simulink model "Air_Conditioner"  (R2016b)
settings: Solver=ode23t  StartTime=0.0  StopTime=24  RelTol=1e-3  EnableMultiTasking=on
model workspace: external: MAT-File (data not in the file)
libraries: simulink x3
settings Model: Creator=jm3gonza  LastModifiedBy=Lenio
settings DataIOCC: SaveFormat=Array  SignalLoggingSaveFormat=ModelDataLogs  SaveState=on
settings OptimizationCC: ExpressionDepthLimit=2147483647  LifeSpan=inf
settings DebuggingCC: AlgebraicLoopMsg=none  UnderspecifiedInitializationDetection=Classic  MergeDetectMultiDrivingBlocksExec=none  FcnCallInpInsideContextMsg=warning  UnconnectedInputMsg=none  UnconnectedOutputMsg=none  UnconnectedLineMsg=none  StateNameClashWarn=warning  SFUnexpectedBacktrackingDiag=warning  SFNoUnconditionalDefaultTransitionDiag=warning  SFExecutionAtInitializationDiag=none
settings HardwareCC: ProdBitPerPointer=32  ProdBitPerSizeT=32  ProdBitPerPtrDiffT=32  ProdLargestAtomicFloat=None  ProdIntDivRoundTo=Undefined  ProdEndianess=Unspecified  ProdWordSize=32  ProdHWDeviceType=32-bit Generic
settings ModelReferenceCC: PropagateSignalLabelsOutOfModel=off
settings GRTTargetCC: TargetLangStandard=C89/C90 (ANSI)  GeneratePreprocessorConditionals=Disable all  CombineOutputUpdateFcns=off  GRTInterface=on
settings ConfigComp: CovMetricSettings=dw  CovHtmlReporting=on  CovSaveCumulativeToWorkspaceVar=on  CovSaveSingleToWorkspaceVar=on  CovExternalEMLEnable=off

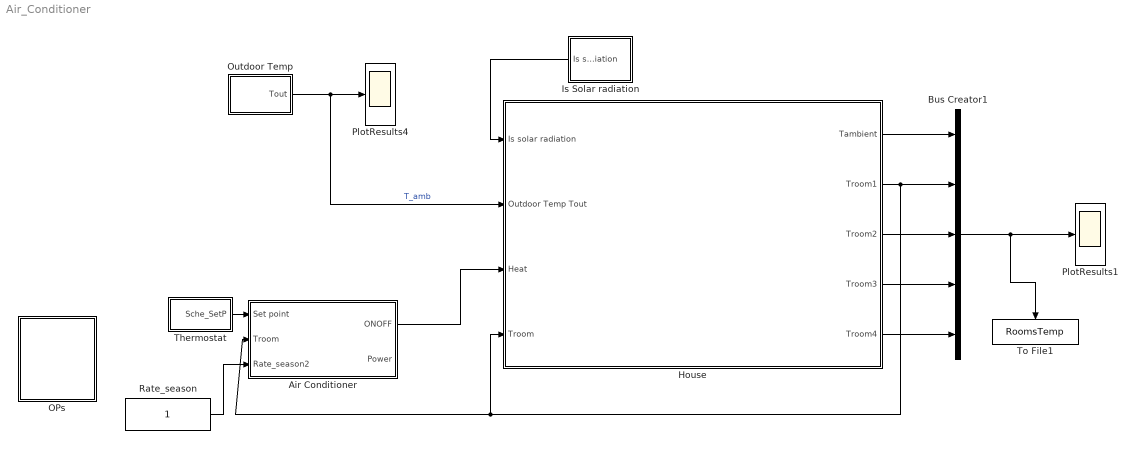
== system Air_Conditioner ==
  Air Conditioner : Subsystem
  Bus Creator1 : BusCreator  Inputs=5
  House : Subsystem
  Is Solar radiation : Subsystem
  OPs : Subsystem
  Outdoor Temp : Subsystem
  PlotResults1 : Scope
  PlotResults4 : Scope
  Rate_season : Constant
  Thermostat : Subsystem
  To File1 : ToFile  Filename=RoomsTemp  MatrixName=RoomsTemp
  wires:
  Outdoor Temp/1(Tout) -> PlotResults4/1, House/2(Outdoor Temp Tout)  "T_amb"
  House/5(Troom4) -> Bus Creator1/5
  House/1(Tambient) -> Bus Creator1/1
  House/2(Troom1) -> Bus Creator1/2, House/4(Troom), Air Conditioner/2(Troom)
  House/3(Troom2) -> Bus Creator1/3
  House/4(Troom3) -> Bus Creator1/4
  Bus Creator1/1 -> To File1/1, PlotResults1/1
  Air Conditioner/1(ONOFF) -> House/3(Heat)
  Is Solar radiation/1(Is solar radiation) -> House/1(Is solar radiation)
  Thermostat/1(Sche_SetP) -> Air Conditioner/1(Set point)
  Rate_season/1 -> Air Conditioner/3(Rate_season2)

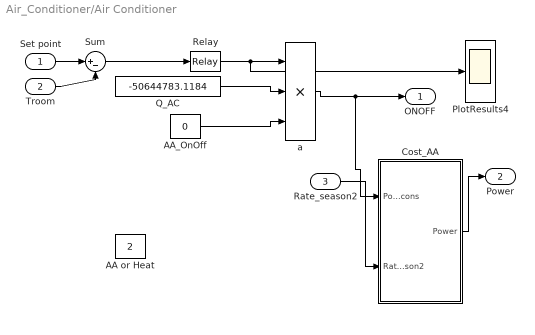
== system Air_Conditioner/Air Conditioner ==
  Set point : Inport
  Troom : Inport  Port=2
  Rate_season2 : Inport  Port=3
  AA or Heat : Constant  Value=2
  AA_OnOff : Constant  Value=0
  Cost_AA : Subsystem
  PlotResults4 : Scope
  Q_AC : Constant  Value=-50644783.1184
  Relay : Relay  OnSwitchValue=0.5  OffSwitchValue=-0.5  OnOutputValue=0  OffOutputValue=1
  Sum : Sum  Inputs=|+-  SampleTime=0  SaturateOnIntegerOverflow=on  InputSameDT=on  OutDataTypeStr=Inherit: Same as first input
  a : Product  Inputs=3  RndMeth=Zero
  ONOFF : Outport  InitialOutput=0
  Power : Outport  Port=2  InitialOutput=0
  wires:
  Set point/1 -> Sum/1
  Troom/1 -> Sum/2
  Sum/1 -> Relay/1
  Relay/1 -> a/1, PlotResults4/1
  a/1 -> ONOFF/1, Cost_AA/1(Powe_cons)
  Q_AC/1 -> a/2
  AA_OnOff/1 -> a/3
  Rate_season2/1 -> Cost_AA/2(Rate_season2)
  Cost_AA/1(Power) -> Power/1

== system Air_Conditioner/House ==
  Is solar radiation : Inport
  Outdoor Temp Tout : Inport  Port=2
  Heat : Inport  Port=3
  Troom : Inport  Port=4
  Room_1 : Subsystem
  Room_2 : Subsystem
  Room_3 : Subsystem
  Room_4 : Subsystem
  Tambient : Outport  InitialOutput=0
  Troom1 : Outport  Port=2  InitialOutput=0
  Troom2 : Outport  Port=3  InitialOutput=0
  Troom3 : Outport  Port=4  InitialOutput=0
  Troom4 : Outport  Port=5  InitialOutput=0
  wires:
  Is solar radiation/1 -> Room_1/1(Is solar radiation), Room_2/1(Is solar radiation), Room_3/1(Is solar radiation), Room_4/1(Is solar radiation)
  Outdoor Temp Tout/1 -> Room_1/2(Outdoor Temp Tout), Room_2/2(Outdoor Temp Tout), Room_3/2(Outdoor Temp Tout), Room_4/2(Outdoor Temp Tout), Tambient/1
  Heat/1 -> Room_1/3(Q_Heat), Room_2/3(Q_Heat), Room_3/3(Q_Heat), Room_4/3(Q_Heat)  "Q_Heat"
  Troom/1 -> Room_1/4(Troom), Room_2/4(Troom), Room_3/4(Troom), Room_4/4(Troom)
  Room_1/1(Room Temp Troom) -> Troom1/1
  Room_2/1(Room Temp Troom) -> Troom2/1
  Room_3/1(Room Temp Troom) -> Troom3/1
  Room_4/1(Room Temp Troom) -> Troom4/1

== system Air_Conditioner/Is Solar radiation ==
  Avg Outdoor Temp : Constant
  Outdoor Temp : simulink/Sources/Repeating Sequence Interpolated  OutValues=|  TimeValues=|  LookUpMeth=Interpolation-Use End Values  tsamp=-1  OutMin=[]  OutMax=[]  OutDataTypeStr=double  OutputDataTypeScalingMode=double  OutDataType=fixdt(0,8)  OutScaling=2^-10
      OutValues=|
      | [0
      | 0
      | 0
      | 0
      | 0
      | 0
      | 0
      | 0
      | 0
      | 0
      | 0
      | 0
      | 0
      | 0
      | 0
      | 0
      | 0
      | 0
      | 0
      | 0
      | 0
      | 12.85
      | 12.85
      | 12.85
      | 25.699
      | 38.55
      | 51.399
      | 38.55
      | 70.673
      | 70.674
      | 122.073
      | 147.772
      | 102.797
      | 237.697
      | 160.597
      | 186.273
      | 186.268
      | 173.422
      | 404.649
      | 571.658
      | 327.556
      | 411.017
      | 468.811
      | 391.717
      | 314.634
      | 237.577
      | 301.802
      | 417.367
      | 584.316
      | 449.469
      | 719.125
      | 532.917
      | 340.26
      | 199.027
      | 340.266
      | 404.503
      | 288.922
      | 314.601
      | 340.296
      | 301.769
      | 288.938
      | 263.253
      | 288.942
      | 321.049
      | 417.349
      | 327.463
      | 365.947
      | 365.936
      | 269.636
      | 224.709
      | 231.145
      | 173.362
      | 154.103
      | 147.682
      | 128.422
      | 102.737
      | 83.473
      | 70.634
      | 25.685
      | 25.686
      | 0
      | 0
      | 0
      | 0
      | 0
      | 0
      | 0
      | 0
      | 0
      | 0
      | 0
      | 0
      | 0
      | 0
      | 0
      | 0
      | ].'
      TimeValues=|
      | [         0
      |     0.1500
      |     0.3000
      |     0.4500
      |     1.0000
      |     1.1500
      |     1.3000
      |     1.4500
      |     2.0000
      |     2.1500
      |     2.3000
      |     2.4500
      |     3.0000
      |     3.1500
      |     3.3000
      |     3.4500
      |     4.0000
      |     4.1500
      |     4.3000
      |     4.4500
      |     5.0000
      |     5.1500
      |     5.3000
      |     5.4500
      |     6.0000
      |     6.1500
      |     6.3000
      |     6.4500
      |     7.0000
      |     7.1500
      |     7.3000
      |     7.4500
      |     8.0000
      |     8.1500
      |     8.3000
      |     8.4500
      |     9.0000
      |     9.1500
      |     9.3000
      |     9.4500
      |    10.0000
      |    10.1500
      |    10.3000
      |    10.4500
      |    11.0000
      |    11.1500
      |    11.3000
      |    11.4500
      |    12.0000
      |    12.1500
      |    12.3000
      |    12.4500
      |    13.0000
      |    13.1500
      |    13.3000
      |    13.4500
      |    14.0000
      |    14.1500
      |    14.3000
      |    14.4500
      |    15.0000
      |    15.1500
      |    15.3000
      |    15.4500
      |    16.0000
      |    16.1500
      |    16.3000
      |    16.4500
      |    17.0000
      |    17.1500
      |    17.3000
      |    17.4500
      |    18.0000
      |    18.1500
      |    18.3000
      |    18.4500
      |    19.0000
      |    19.1500
      |    19.3000
      |    19.4500
      |    20.0000
      |    20.1500
      |    20.3000
      |    20.4500
      |    21.0000
      |    21.1500
      |    21.3000
      |    21.4500
      |    22.0000
      |    22.1500
      |    22.3000
      |    22.4500
      |    23.0000
      |    23.1500
      |    23.3000
      |    23.4500].'
  Sum1 : Sum  Inputs=|++  SaturateOnIntegerOverflow=on  InputSameDT=on  OutDataTypeStr=Inherit: Same as first input
  Is solar radiation : Outport  InitialOutput=0
  wires:
  Avg Outdoor Temp/1 -> Sum1/1
  Outdoor Temp/1 -> Sum1/2
  Sum1/1 -> Is solar radiation/1

== system Air_Conditioner/OPs ==
  Bus Creator : BusCreator  Inputs=6
  Dishwasher_OP : Constant  Value=0
  Dryer_OP : Constant  Value=0
  EveryOP : Constant
  Lighting_OP : Constant  Value=0
  Stove_OP : Constant  Value=0
  Terminator : Terminator
  Washer_OP : Constant  Value=0
  wires:
  Lighting_OP/1 -> Bus Creator/2
  Dryer_OP/1 -> Bus Creator/3
  Dishwasher_OP/1 -> Bus Creator/4
  Washer_OP/1 -> Bus Creator/5
  EveryOP/1 -> Bus Creator/6
  Stove_OP/1 -> Bus Creator/1
  Bus Creator/1 -> Terminator/1

== system Air_Conditioner/Outdoor Temp ==
  Heater Switch1 : Product  RndMeth=Zero
  Heater Switch2 : Product  RndMeth=Zero
  Sum2 : Sum  SaturateOnIntegerOverflow=on  InputSameDT=on  OutDataTypeStr=Inherit: Same as first input
  Summer : simulink/Sources/Repeating Sequence Interpolated  OutValues=|  TimeValues=|  LookUpMeth=Interpolation-Use End Values  tsamp=-1  OutMin=[]  OutMax=[]  OutDataTypeStr=double  OutputDataTypeScalingMode=double  OutDataType=fixdt(0,8)  OutScaling=2^-10
      OutValues=|
      | [   23.8160
      |    23.7130
      |    23.4480
      |    23.2590
      |    23.1710
      |    23.1330
      |    22.9330
      |    22.8600
      |    22.7100
      |    22.6330
      |    22.4980
      |    22.3130
      |    22.2390
      |    22.1040
      |    21.9830
      |    21.7030
      |    21.5360
      |    21.4650
      |    21.8150
      |    22.1730
      |    22.3830
      |    22.6540
      |    22.7390
      |    22.9630
      |    23.3760
      |    23.9600
      |    24.3460
      |    24.7420
      |    24.9870
      |    25.3280
      |    25.6220
      |    26.4600
      |    26.8940
      |    27.7100
      |    27.9620
      |    28.1630
      |    28.4950
      |    29.0620
      |    29.0190
      |    29.0170
      |    29.2500
      |    29.6940
      |    29.8860
      |    29.9560
      |    30.0730
      |    30.6760
      |    30.8120
      |    30.9150
      |    31.2920
      |    30.8100
      |    31.3250
      |    31.3570
      |    31.6710
      |    32.3710
      |    31.6010
      |    32.0310
      |    32.1090
      |    32.3180
      |    32.3980
      |    31.7870
      |    31.6290
      |    33.0060
      |    33.0040
      |    32.8570
      |    32.9240
      |    32.6620
      |    33.1210
      |    32.6940
      |    32.3640
      |    32.0100
      |    31.5350
      |    32.0310
      |    31.0020
      |    30.4620
      |    30.0880
      |    29.8870
      |    29.5410
      |    29.3690
      |    29.1040
      |    28.6390
      |    28.1200
      |    26.7970
      |    26.0180
      |    25.6170
      |    26.9460
      |    27.3140
      |    27.1220
      |    26.8170
      |    26.5690
      |    26.4040
      |    26.2680
      |    26.1190
      |    25.7690
      |    25.4730
      |    25.2080
      |    24.9570].'
      TimeValues=|
      | [         0
      |     0.1500
      |     0.3000
      |     0.4500
      |     1.0000
      |     1.1500
      |     1.3000
      |     1.4500
      |     2.0000
      |     2.1500
      |     2.3000
      |     2.4500
      |     3.0000
      |     3.1500
      |     3.3000
      |     3.4500
      |     4.0000
      |     4.1500
      |     4.3000
      |     4.4500
      |     5.0000
      |     5.1500
      |     5.3000
      |     5.4500
      |     6.0000
      |     6.1500
      |     6.3000
      |     6.4500
      |     7.0000
      |     7.1500
      |     7.3000
      |     7.4500
      |     8.0000
      |     8.1500
      |     8.3000
      |     8.4500
      |     9.0000
      |     9.1500
      |     9.3000
      |     9.4500
      |    10.0000
      |    10.1500
      |    10.3000
      |    10.4500
      |    11.0000
      |    11.1500
      |    11.3000
      |    11.4500
      |    12.0000
      |    12.1500
      |    12.3000
      |    12.4500
      |    13.0000
      |    13.1500
      |    13.3000
      |    13.4500
      |    14.0000
      |    14.1500
      |    14.3000
      |    14.4500
      |    15.0000
      |    15.1500
      |    15.3000
      |    15.4500
      |    16.0000
      |    16.1500
      |    16.3000
      |    16.4500
      |    17.0000
      |    17.1500
      |    17.3000
      |    17.4500
      |    18.0000
      |    18.1500
      |    18.3000
      |    18.4500
      |    19.0000
      |    19.1500
      |    19.3000
      |    19.4500
      |    20.0000
      |    20.1500
      |    20.3000
      |    20.4500
      |    21.0000
      |    21.1500
      |    21.3000
      |    21.4500
      |    22.0000
      |    22.1500
      |    22.3000
      |    22.4500
      |    23.0000
      |    23.1500
      |    23.3000
      |    23.4500].'
  Temp_aux : Constant  SampleTime=0
  Temp_aux1 : Constant  Value=0  SampleTime=0
  Winter : simulink/Sources/Repeating Sequence Interpolated  OutValues=|  TimeValues=|  LookUpMeth=Interpolation-Use End Values  tsamp=-1  OutMin=[]  OutMax=[]  OutDataTypeStr=double  OutputDataTypeScalingMode=double  OutDataType=fixdt(0,8)  OutScaling=2^-10
      OutValues=|
      | [  -11.1291
      |   -11.1588
      |   -11.2754
      |   -11.3348
      |   -11.3640
      |   -11.3349
      |   -11.2761
      |   -11.3644
      |   -11.4820
      |   -11.6877
      |   -11.9824
      |   -12.3084
      |   -12.4564
      |   -12.7586
      |   -12.9110
      |   -13.1851
      |   -13.3978
      |   -13.7036
      |   -13.6713
      |   -14.1054
      |   -13.8875
      |   -13.7327
      |   -13.6400
      |   -13.6400
      |   -13.7636
      |   -13.8879
      |   -14.1072
      |   -14.3577
      |   -14.5135
      |   -14.6391
      |   -14.6391
      |   -14.3243
      |   -14.2618
      |   -14.0769
      |   -13.3678
      |   -13.1847
      |   -13.1874
      |   -12.8845
      |   -12.1952
      |   -12.1968
      |   -11.7508
      |   -11.6376
      |   -11.1100
      |   -10.7030
      |   -10.1258
      |    -9.5609
      |    -9.5616
      |    -9.1089
      |    -8.8274
      |    -8.6038
      |    -8.0754
      |    -7.9926
      |    -7.0311
      |    -6.4872
      |    -6.3536
      |    -6.0586
      |    -5.7638
      |    -5.5768
      |    -5.2566
      |    -5.2045
      |    -4.5670
      |    -3.8272
      |    -3.7990
      |    -3.8776
      |    -3.7724
      |    -3.8777
      |    -4.3791
      |    -4.7245
      |    -4.5643
      |    -4.8546
      |    -5.4121
      |    -5.8135
      |    -6.1916
      |    -6.5106
      |    -6.7813
      |    -7.1642
      |    -7.2707
      |    -7.4860
      |    -7.6777
      |    -7.7616
      |    -8.1494
      |    -8.2612
      |    -9.1811
      |    -9.5460
      |   -10.2024
      |   -10.1740
      |   -10.7173
      |   -11.6519
      |   -11.9196
      |   -13.5221
      |   -14.0461
      |   -14.9577
      |   -15.4698
      |   -15.7285
      |   -16.0525
      |   -16.2152
      |   -16.2152
      |   -16.52].'
      TimeValues=|
      | [         0
      |     0.1500
      |     0.3000
      |     0.4500
      |     1.0000
      |     1.1500
      |     1.3000
      |     1.4500
      |     2.0000
      |     2.1500
      |     2.3000
      |     2.4500
      |     3.0000
      |     3.1500
      |     3.3000
      |     3.4500
      |     4.0000
      |     4.1500
      |     4.3000
      |     4.4500
      |     5.0000
      |     5.1500
      |     5.3000
      |     5.4500
      |     6.0000
      |     6.1500
      |     6.3000
      |     6.4500
      |     7.0000
      |     7.1500
      |     7.3000
      |     7.4500
      |     8.0000
      |     8.1500
      |     8.3000
      |     8.4500
      |     9.0000
      |     9.1500
      |     9.3000
      |     9.4500
      |    10.0000
      |    10.1500
      |    10.3000
      |    10.4500
      |    11.0000
      |    11.1500
      |    11.3000
      |    11.4500
      |    12.0000
      |    12.1500
      |    12.3000
      |    12.4500
      |    13.0000
      |    13.1500
      |    13.3000
      |    13.4500
      |    14.0000
      |    14.1500
      |    14.3000
      |    14.4500
      |    15.0000
      |    15.1500
      |    15.3000
      |    15.4500
      |    16.0000
      |    16.1500
      |    16.3000
      |    16.4500
      |    17.0000
      |    17.1500
      |    17.3000
      |    17.4500
      |    18.0000
      |    18.1500
      |    18.3000
      |    18.4500
      |    19.0000
      |    19.1500
      |    19.3000
      |    19.4500
      |    20.0000
      |    20.1500
      |    20.3000
      |    20.4500
      |    21.0000
      |    21.1500
      |    21.3000
      |    21.4500
      |    22.0000
      |    22.1500
      |    22.3000
      |    22.4500
      |    23.0000
      |    23.1500
      |    23.3000
      |    23.4500
      |    23.900  
      |    24.000].'
  Tout : Outport  InitialOutput=0
  wires:
  Heater Switch1/1 -> Sum2/1  "Toutdoors"
  Temp_aux/1 -> Heater Switch1/1
  Summer/1 -> Heater Switch1/2
  Heater Switch2/1 -> Sum2/2  "Toutdoors"
  Temp_aux1/1 -> Heater Switch2/1
  Winter/1 -> Heater Switch2/2
  Sum2/1 -> Tout/1

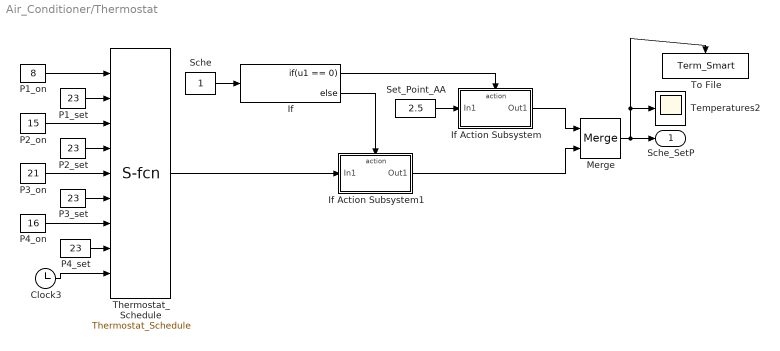
== system Air_Conditioner/Thermostat ==
  Clock3 : Clock
      settings: Decimation=100
  If : If  IfExpression=u1 == 0
  If Action Subsystem : Subsystem  TreatAsAtomicUnit=on
  If Action Subsystem1 : Subsystem  TreatAsAtomicUnit=on
  Merge : Merge
  P1_on : Constant  Value=8
  P1_set : Constant  Value=23
  P2_on : Constant  Value=15
  P2_set : Constant  Value=23
  P3_on : Constant  Value=21
  P3_set : Constant  Value=23
  P4_on : Constant  Value=16
  P4_set : Constant  Value=23
  Sche : Constant
  Set_Point_AA : Constant  Value=2.5
  Temperatures2 : Scope
  Thermostat_Schedule : M-S-Function  FunctionName=Thermostat_Schedule
  To File : ToFile  Filename=Term_Smart  MatrixName=Term_Smart
  Sche_SetP : Outport  InitialOutput=0
  wires:
  P1_on/1 -> Thermostat_Schedule/1
  P1_set/1 -> Thermostat_Schedule/2
  P2_on/1 -> Thermostat_Schedule/3
  P2_set/1 -> Thermostat_Schedule/4
  P3_on/1 -> Thermostat_Schedule/5
  P3_set/1 -> Thermostat_Schedule/6
  P4_on/1 -> Thermostat_Schedule/7
  P4_set/1 -> Thermostat_Schedule/8
  Clock3/1 -> Thermostat_Schedule/9
  Sche/1 -> If/1
  If/1 -> If Action Subsystem/Action
  Set_Point_AA/1 -> If Action Subsystem/1(In1)
  If/2 -> If Action Subsystem1/Action
  Merge/1 -> Sche_SetP/1, Temperatures2/1, To File/1
  Thermostat_Schedule/1 -> If Action Subsystem1/1(In1)
  If Action Subsystem1/1(Out1) -> Merge/2
  If Action Subsystem/1(Out1) -> Merge/1

== system Air_Conditioner/Air Conditioner/Cost_AA ==
  Powe_cons : Inport
  Rate_season2 : Inport  Port=2
  AcHt : Gain  SaturateOnIntegerOverflow=on  OutDataTypeStr=Inherit: Same as input  ParamDataTypeStr=Inherit: Same as input
  Bus Creator2 : BusCreator  Inputs=3
  Integrator : Integrator
  Integrator3 : Integrator
  PlotResults1 : Scope
  PlotResults2 : Scope
  PlotResults4 : Scope
  Rates : Subsystem
  To File : ToFile  Filename=Pow_Cost_AC  MatrixName=Pow_Cost_AC
  Watts-->kW : Gain  Gain=-1/(3600*1000)  SaturateOnIntegerOverflow=on  OutDataTypeStr=Inherit: Same as input  ParamDataTypeStr=Inherit: Same as input
  Power : Outport  InitialOutput=0
  wires:
  Rates/1(Rate) -> Integrator/1
  Integrator3/1 -> Bus Creator2/2  "kw_hr"
  Bus Creator2/1 -> To File/1, PlotResults1/1
  Integrator/1 -> PlotResults2/1, Bus Creator2/3  "Cost_hr"
  Watts-->kW/1 -> Integrator3/1, Bus Creator2/1, PlotResults4/1, Rates/1(Powe_cons), Power/1
  AcHt/1 -> Watts-->kW/1
  Powe_cons/1 -> AcHt/1
  Rate_season2/1 -> Rates/2(Rate_season2)

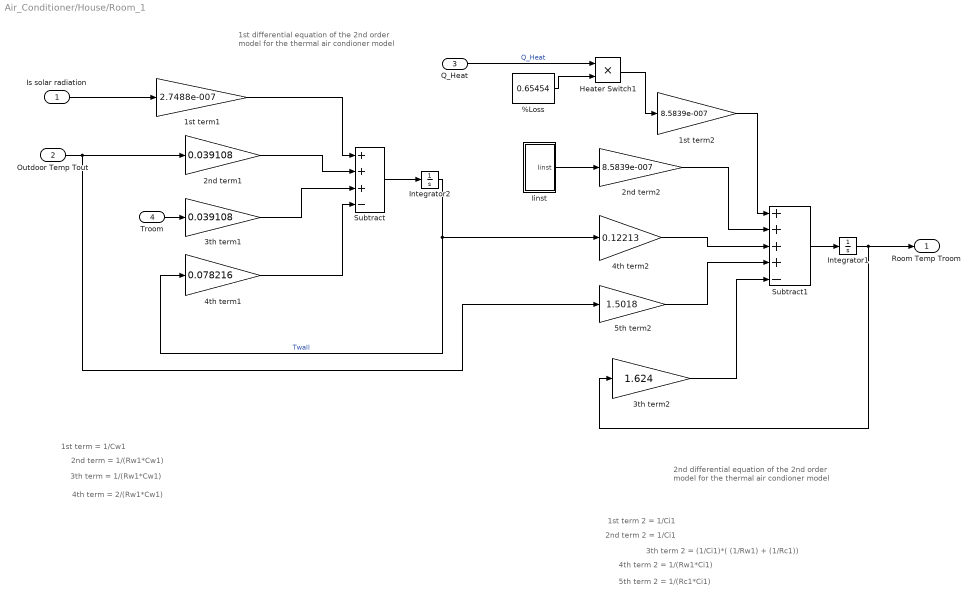
== system Air_Conditioner/House/Room_1 ==
  note: 1st differential equation of the 2nd order
      | model for the thermal air condioner model
  note: 2nd differential equation of the 2nd order
      | model for the thermal air condioner model
  note: 1st term = 1/Cw1
  note: 2nd term = 1/(Rw1*Cw1)
  note: 3th term = 1/(Rw1*Cw1)
  note: 4th term = 2/(Rw1*Cw1)
  note: 1st term 2 = 1/Ci1
  note: 2nd term 2 = 1/Ci1
  note: 3th term 2 = (1/Ci1)*( (1/Rw1) + (1/Rc1))
  note: 4th term 2 = 1/(Rw1*Ci1)
  note: 5th term 2 = 1/(Rc1*Ci1)
  Is solar radiation : Inport
  Outdoor Temp Tout : Inport  Port=2
  Q_Heat : Inport  Port=3
  Troom : Inport  Port=4
  %Loss : Constant  Value=0.65454
  1st term1 : Gain  Gain=2.7488e-007
  1st term2 : Gain  Gain=8.5839e-007
  2nd term1 : Gain  Gain=0.039108
  2nd term2 : Gain  Gain=8.5839e-007
  3th term1 : Gain  Gain=0.039108
  3th term2 : Gain  Gain=1.624
  4th term1 : Gain  Gain=0.078216
  4th term2 : Gain  Gain=0.12213
  5th term2 : Gain  Gain=1.5018
  Heater Switch1 : Product  RndMeth=Zero
  Iinst : Subsystem
  Integrator1 : Integrator  InitialCondition=21
  Integrator2 : Integrator  InitialCondition=21
  Subtract : Sum  Inputs=+++-
  Subtract1 : Sum  Inputs=++++-
  Room Temp Troom : Outport  InitialOutput=0
  wires:
  2nd term1/1 -> Subtract/2
  4th term1/1 -> Subtract/4
  Subtract/1 -> Integrator2/1
  Integrator2/1 -> 4th term1/1, 4th term2/1  "Twall"
  Integrator1/1 -> 3th term2/1, Room Temp Troom/1
  Subtract1/1 -> Integrator1/1
  Outdoor Temp Tout/1 -> 2nd term1/1, 5th term2/1
  Troom/1 -> 3th term1/1
  3th term1/1 -> Subtract/3
  1st term1/1 -> Subtract/1
  2nd term2/1 -> Subtract1/2
  Iinst/1(Iinst) -> 2nd term2/1
  Is solar radiation/1 -> 1st term1/1
  4th term2/1 -> Subtract1/3
  5th term2/1 -> Subtract1/4
  3th term2/1 -> Subtract1/5
  Q_Heat/1 -> Heater Switch1/1  "Q_Heat"
  %Loss/1 -> Heater Switch1/2
  1st term2/1 -> Subtract1/1
  Heater Switch1/1 -> 1st term2/1

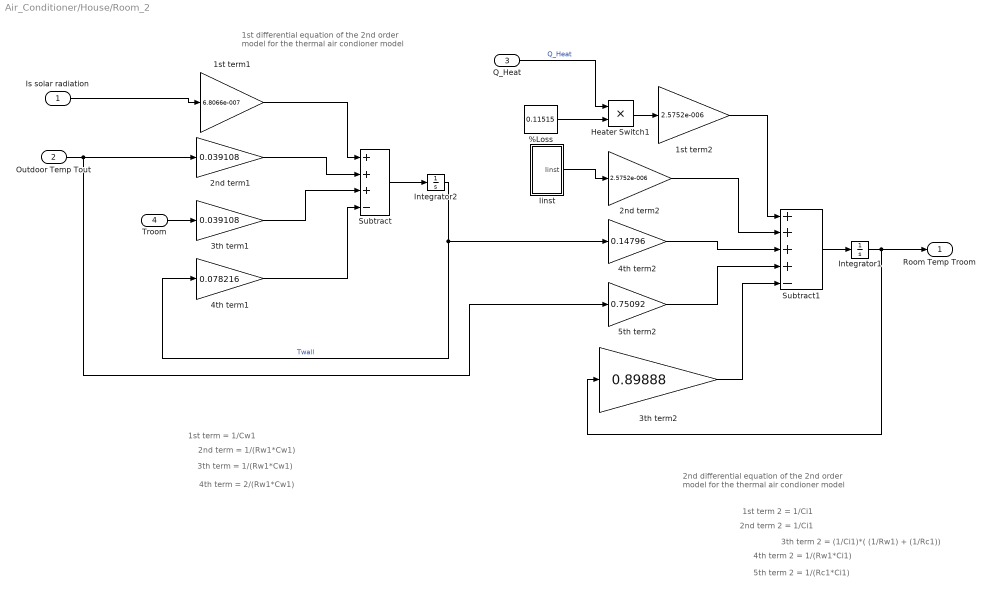
== system Air_Conditioner/House/Room_2 ==
  note: 1st differential equation of the 2nd order
      | model for the thermal air condioner model
  note: 2nd differential equation of the 2nd order
      | model for the thermal air condioner model
  note: 1st term = 1/Cw1
  note: 2nd term = 1/(Rw1*Cw1)
  note: 3th term = 1/(Rw1*Cw1)
  note: 4th term = 2/(Rw1*Cw1)
  note: 1st term 2 = 1/Ci1
  note: 2nd term 2 = 1/Ci1
  note: 3th term 2 = (1/Ci1)*( (1/Rw1) + (1/Rc1))
  note: 4th term 2 = 1/(Rw1*Ci1)
  note: 5th term 2 = 1/(Rc1*Ci1)
  Is solar radiation : Inport
  Outdoor Temp Tout : Inport  Port=2
  Q_Heat : Inport  Port=3
  Troom : Inport  Port=4
  %Loss : Constant  Value=0.11515
  1st term1 : Gain  Gain=6.8066e-007
  1st term2 : Gain  Gain=2.5752e-006
  2nd term1 : Gain  Gain=0.039108
  2nd term2 : Gain  Gain=2.5752e-006
  3th term1 : Gain  Gain=0.039108
  3th term2 : Gain  Gain=0.89888
  4th term1 : Gain  Gain=0.078216
  4th term2 : Gain  Gain=0.14796
  5th term2 : Gain  Gain=0.75092
  Heater Switch1 : Product  RndMeth=Zero
  Iinst : Subsystem
  Integrator1 : Integrator  InitialCondition=21
  Integrator2 : Integrator  InitialCondition=21
  Subtract : Sum  Inputs=+++-
  Subtract1 : Sum  Inputs=++++-
  Room Temp Troom : Outport  InitialOutput=0
  wires:
  2nd term1/1 -> Subtract/2
  4th term1/1 -> Subtract/4
  Subtract/1 -> Integrator2/1
  Integrator2/1 -> 4th term1/1, 4th term2/1  "Twall"
  Integrator1/1 -> 3th term2/1, Room Temp Troom/1
  Subtract1/1 -> Integrator1/1
  Outdoor Temp Tout/1 -> 2nd term1/1, 5th term2/1
  Troom/1 -> 3th term1/1
  3th term1/1 -> Subtract/3
  1st term1/1 -> Subtract/1
  2nd term2/1 -> Subtract1/2
  Q_Heat/1 -> Heater Switch1/1  "Q_Heat"
  Iinst/1(Iinst) -> 2nd term2/1
  Is solar radiation/1 -> 1st term1/1
  4th term2/1 -> Subtract1/3
  5th term2/1 -> Subtract1/4
  3th term2/1 -> Subtract1/5
  %Loss/1 -> Heater Switch1/2
  Heater Switch1/1 -> 1st term2/1
  1st term2/1 -> Subtract1/1

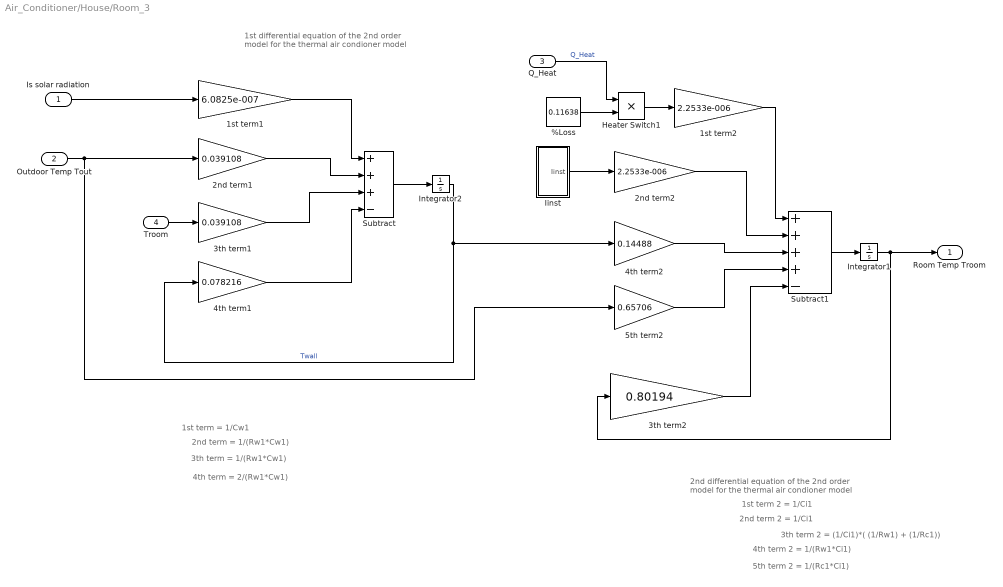
== system Air_Conditioner/House/Room_3 ==
  note: 1st differential equation of the 2nd order
      | model for the thermal air condioner model
  note: 2nd differential equation of the 2nd order
      | model for the thermal air condioner model
  note: 1st term = 1/Cw1
  note: 2nd term = 1/(Rw1*Cw1)
  note: 3th term = 1/(Rw1*Cw1)
  note: 4th term = 2/(Rw1*Cw1)
  note: 1st term 2 = 1/Ci1
  note: 2nd term 2 = 1/Ci1
  note: 3th term 2 = (1/Ci1)*( (1/Rw1) + (1/Rc1))
  note: 4th term 2 = 1/(Rw1*Ci1)
  note: 5th term 2 = 1/(Rc1*Ci1)
  Is solar radiation : Inport
  Outdoor Temp Tout : Inport  Port=2
  Q_Heat : Inport  Port=3
  Troom : Inport  Port=4
  %Loss : Constant  Value=0.11638
  1st term1 : Gain  Gain=6.0825e-007
  1st term2 : Gain  Gain=2.2533e-006
  2nd term1 : Gain  Gain=0.039108
  2nd term2 : Gain  Gain=2.2533e-006
  3th term1 : Gain  Gain=0.039108
  3th term2 : Gain  Gain=0.80194
  4th term1 : Gain  Gain=0.078216
  4th term2 : Gain  Gain=0.14488
  5th term2 : Gain  Gain=0.65706
  Heater Switch1 : Product  RndMeth=Zero
  Iinst : Subsystem
  Integrator1 : Integrator  InitialCondition=21
  Integrator2 : Integrator  InitialCondition=21
  Subtract : Sum  Inputs=+++-
  Subtract1 : Sum  Inputs=++++-
  Room Temp Troom : Outport  InitialOutput=0
  wires:
  2nd term1/1 -> Subtract/2
  4th term1/1 -> Subtract/4
  Subtract/1 -> Integrator2/1
  Integrator2/1 -> 4th term1/1, 4th term2/1  "Twall"
  Integrator1/1 -> 3th term2/1, Room Temp Troom/1
  Subtract1/1 -> Integrator1/1
  Outdoor Temp Tout/1 -> 2nd term1/1, 5th term2/1
  Troom/1 -> 3th term1/1
  3th term1/1 -> Subtract/3
  1st term1/1 -> Subtract/1
  2nd term2/1 -> Subtract1/2
  Q_Heat/1 -> Heater Switch1/1  "Q_Heat"
  Iinst/1(Iinst) -> 2nd term2/1
  Is solar radiation/1 -> 1st term1/1
  4th term2/1 -> Subtract1/3
  5th term2/1 -> Subtract1/4
  3th term2/1 -> Subtract1/5
  %Loss/1 -> Heater Switch1/2
  1st term2/1 -> Subtract1/1
  Heater Switch1/1 -> 1st term2/1

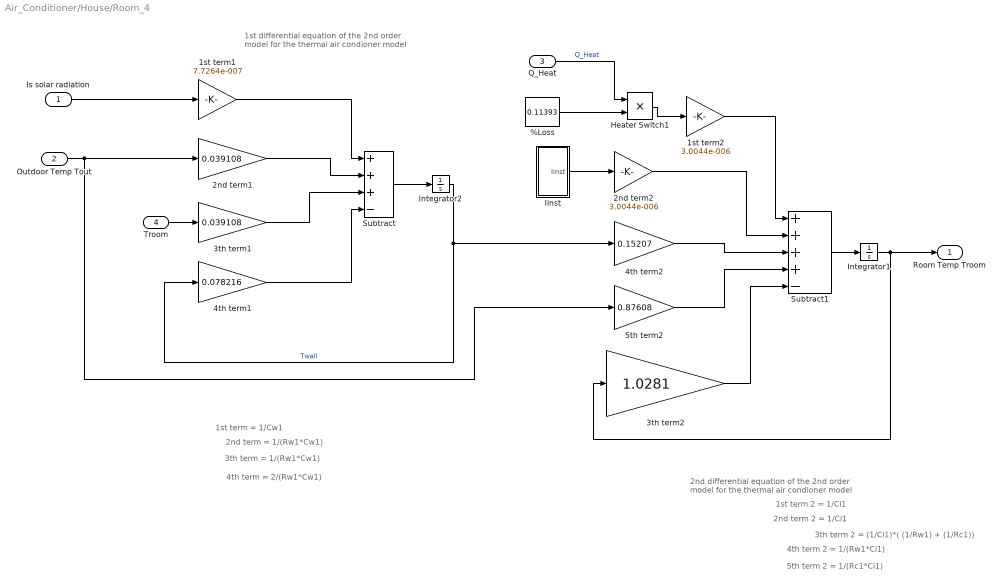
== system Air_Conditioner/House/Room_4 ==
  note: 1st differential equation of the 2nd order
      | model for the thermal air condioner model
  note: 2nd differential equation of the 2nd order
      | model for the thermal air condioner model
  note: 1st term = 1/Cw1
  note: 2nd term = 1/(Rw1*Cw1)
  note: 3th term = 1/(Rw1*Cw1)
  note: 4th term = 2/(Rw1*Cw1)
  note: 1st term 2 = 1/Ci1
  note: 2nd term 2 = 1/Ci1
  note: 3th term 2 = (1/Ci1)*( (1/Rw1) + (1/Rc1))
  note: 4th term 2 = 1/(Rw1*Ci1)
  note: 5th term 2 = 1/(Rc1*Ci1)
  Is solar radiation : Inport
  Outdoor Temp Tout : Inport  Port=2
  Q_Heat : Inport  Port=3
  Troom : Inport  Port=4
  %Loss : Constant  Value=0.11393
  1st term1 : Gain  Gain=7.7264e-007
  1st term2 : Gain  Gain=3.0044e-006
  2nd term1 : Gain  Gain=0.039108
  2nd term2 : Gain  Gain=3.0044e-006
  3th term1 : Gain  Gain=0.039108
  3th term2 : Gain  Gain=1.0281
  4th term1 : Gain  Gain=0.078216
  4th term2 : Gain  Gain=0.15207
  5th term2 : Gain  Gain=0.87608
  Heater Switch1 : Product  RndMeth=Zero
  Iinst : Subsystem
  Integrator1 : Integrator  InitialCondition=21
  Integrator2 : Integrator  InitialCondition=21
  Subtract : Sum  Inputs=+++-
  Subtract1 : Sum  Inputs=++++-
  Room Temp Troom : Outport  InitialOutput=0
  wires:
  2nd term1/1 -> Subtract/2
  4th term1/1 -> Subtract/4
  Subtract/1 -> Integrator2/1
  Integrator2/1 -> 4th term1/1, 4th term2/1  "Twall"
  Integrator1/1 -> 3th term2/1, Room Temp Troom/1
  Subtract1/1 -> Integrator1/1
  Outdoor Temp Tout/1 -> 2nd term1/1, 5th term2/1
  Troom/1 -> 3th term1/1
  3th term1/1 -> Subtract/3
  1st term1/1 -> Subtract/1
  2nd term2/1 -> Subtract1/2
  Q_Heat/1 -> Heater Switch1/1  "Q_Heat"
  Iinst/1(Iinst) -> 2nd term2/1
  Is solar radiation/1 -> 1st term1/1
  4th term2/1 -> Subtract1/3
  5th term2/1 -> Subtract1/4
  3th term2/1 -> Subtract1/5
  %Loss/1 -> Heater Switch1/2
  Heater Switch1/1 -> 1st term2/1
  1st term2/1 -> Subtract1/1

== system Air_Conditioner/Thermostat/If Action Subsystem ==
  In1 : Inport
  Action Port : ActionPort  ActionType=then
  Out1 : Outport
  wires:
  In1/1 -> Out1/1

== system Air_Conditioner/Thermostat/If Action Subsystem1 ==
  In1 : Inport
  Action Port : ActionPort  ActionType=else
  Out1 : Outport
  wires:
  In1/1 -> Out1/1

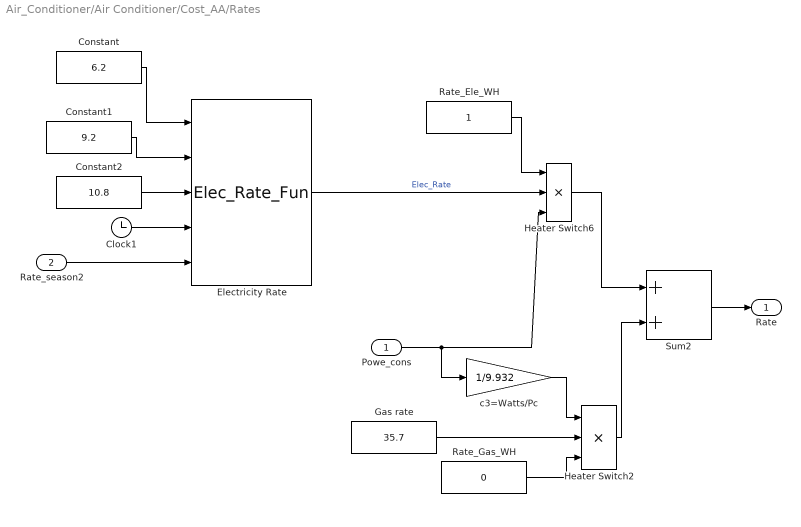
== system Air_Conditioner/Air Conditioner/Cost_AA/Rates ==
  Powe_cons : Inport
  Rate_season2 : Inport  Port=2
  Clock1 : Clock
      settings: Decimation=100
  Constant : Constant  Value=6.2
  Constant1 : Constant  Value=9.2
  Constant2 : Constant  Value=10.8
  Electricity Rate : M-S-Function  FunctionName=Elec_Rate_Fun
  Gas rate : Constant  Value=35.7
  Heater Switch2 : Product  Inputs=3  RndMeth=Zero
  Heater Switch6 : Product  Inputs=3  RndMeth=Zero
  Rate_Ele_WH : Constant
  Rate_Gas_WH : Constant  Value=0
  Sum2 : Sum  SaturateOnIntegerOverflow=on  InputSameDT=on  OutDataTypeStr=Inherit: Same as first input
  c3=Watts/Pc : Gain  Gain=1/9.932  SaturateOnIntegerOverflow=on  OutDataTypeStr=Inherit: Same as input  ParamDataTypeStr=Inherit: Same as input
  Rate : Outport  InitialOutput=0
  wires:
  Constant/1 -> Electricity Rate/1
  Constant1/1 -> Electricity Rate/2
  Constant2/1 -> Electricity Rate/3
  Clock1/1 -> Electricity Rate/4
  Rate_season2/1 -> Electricity Rate/5
  Rate_Ele_WH/1 -> Heater Switch6/1
  Powe_cons/1 -> c3=Watts/Pc/1, Heater Switch6/3
  c3=Watts/Pc/1 -> Heater Switch2/1
  Gas rate/1 -> Heater Switch2/2
  Rate_Gas_WH/1 -> Heater Switch2/3
  Heater Switch6/1 -> Sum2/1
  Heater Switch2/1 -> Sum2/2
  Sum2/1 -> Rate/1
  Electricity Rate/1 -> Heater Switch6/2  "Elec_Rate"

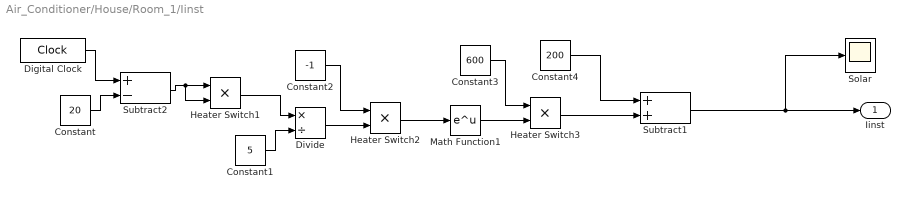
== system Air_Conditioner/House/Room_1/Iinst ==
  Constant : Constant  Value=20
  Constant1 : Constant  Value=5
  Constant2 : Constant  Value=-1
  Constant3 : Constant  Value=600
  Constant4 : Constant  Value=200
  Digital Clock : DigitalClock
  Divide : Product  Inputs=*/
  Heater Switch1 : Product  RndMeth=Zero
  Heater Switch2 : Product  RndMeth=Zero
  Heater Switch3 : Product  RndMeth=Zero
  Math Function1 : Math  SaturateOnIntegerOverflow=on
  Solar : Scope
  Subtract1 : Sum
  Subtract2 : Sum  Inputs=+-
  Iinst : Outport  InitialOutput=0
  wires:
  Digital Clock/1 -> Subtract2/1
  Constant/1 -> Subtract2/2
  Subtract2/1 -> Heater Switch1/1, Heater Switch1/2
  Heater Switch1/1 -> Divide/1
  Constant1/1 -> Divide/2
  Divide/1 -> Heater Switch2/2
  Constant2/1 -> Heater Switch2/1
  Heater Switch2/1 -> Math Function1/1
  Math Function1/1 -> Heater Switch3/2
  Constant3/1 -> Heater Switch3/1
  Subtract1/1 -> Iinst/1, Solar/1
  Constant4/1 -> Subtract1/1
  Heater Switch3/1 -> Subtract1/2

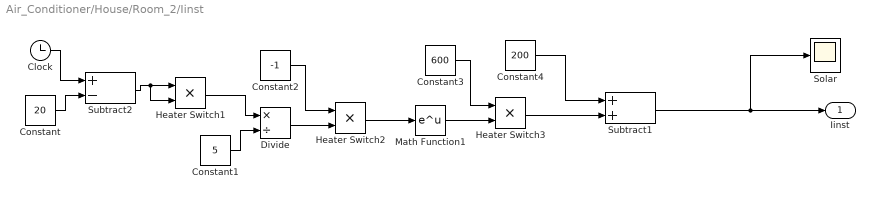
== system Air_Conditioner/House/Room_2/Iinst ==
  Clock : Clock
  Constant : Constant  Value=20
  Constant1 : Constant  Value=5
  Constant2 : Constant  Value=-1
  Constant3 : Constant  Value=600
  Constant4 : Constant  Value=200
  Divide : Product  Inputs=*/
  Heater Switch1 : Product  RndMeth=Zero
  Heater Switch2 : Product  RndMeth=Zero
  Heater Switch3 : Product  RndMeth=Zero
  Math Function1 : Math  SaturateOnIntegerOverflow=on
  Solar : Scope
  Subtract1 : Sum
  Subtract2 : Sum  Inputs=+-
  Iinst : Outport  InitialOutput=0
  wires:
  Clock/1 -> Subtract2/1
  Constant/1 -> Subtract2/2
  Subtract2/1 -> Heater Switch1/1, Heater Switch1/2
  Heater Switch1/1 -> Divide/1
  Constant1/1 -> Divide/2
  Divide/1 -> Heater Switch2/2
  Constant2/1 -> Heater Switch2/1
  Heater Switch2/1 -> Math Function1/1
  Math Function1/1 -> Heater Switch3/2
  Constant3/1 -> Heater Switch3/1
  Subtract1/1 -> Iinst/1, Solar/1
  Constant4/1 -> Subtract1/1
  Heater Switch3/1 -> Subtract1/2

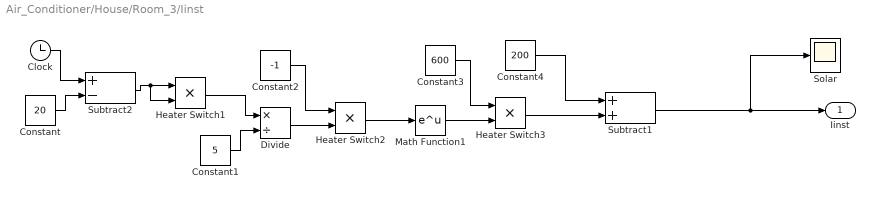
== system Air_Conditioner/House/Room_3/Iinst ==
  Clock : Clock
  Constant : Constant  Value=20
  Constant1 : Constant  Value=5
  Constant2 : Constant  Value=-1
  Constant3 : Constant  Value=600
  Constant4 : Constant  Value=200
  Divide : Product  Inputs=*/
  Heater Switch1 : Product  RndMeth=Zero
  Heater Switch2 : Product  RndMeth=Zero
  Heater Switch3 : Product  RndMeth=Zero
  Math Function1 : Math  SaturateOnIntegerOverflow=on
  Solar : Scope
  Subtract1 : Sum
  Subtract2 : Sum  Inputs=+-
  Iinst : Outport  InitialOutput=0
  wires:
  Clock/1 -> Subtract2/1
  Constant/1 -> Subtract2/2
  Subtract2/1 -> Heater Switch1/1, Heater Switch1/2
  Heater Switch1/1 -> Divide/1
  Constant1/1 -> Divide/2
  Divide/1 -> Heater Switch2/2
  Constant2/1 -> Heater Switch2/1
  Heater Switch2/1 -> Math Function1/1
  Math Function1/1 -> Heater Switch3/2
  Constant3/1 -> Heater Switch3/1
  Subtract1/1 -> Iinst/1, Solar/1
  Constant4/1 -> Subtract1/1
  Heater Switch3/1 -> Subtract1/2

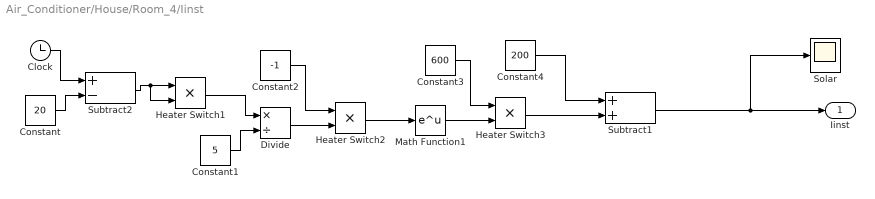
== system Air_Conditioner/House/Room_4/Iinst ==
  Clock : Clock
  Constant : Constant  Value=20
  Constant1 : Constant  Value=5
  Constant2 : Constant  Value=-1
  Constant3 : Constant  Value=600
  Constant4 : Constant  Value=200
  Divide : Product  Inputs=*/
  Heater Switch1 : Product  RndMeth=Zero
  Heater Switch2 : Product  RndMeth=Zero
  Heater Switch3 : Product  RndMeth=Zero
  Math Function1 : Math  SaturateOnIntegerOverflow=on
  Solar : Scope
  Subtract1 : Sum
  Subtract2 : Sum  Inputs=+-
  Iinst : Outport  InitialOutput=0
  wires:
  Clock/1 -> Subtract2/1
  Constant/1 -> Subtract2/2
  Subtract2/1 -> Heater Switch1/1, Heater Switch1/2
  Heater Switch1/1 -> Divide/1
  Constant1/1 -> Divide/2
  Divide/1 -> Heater Switch2/2
  Constant2/1 -> Heater Switch2/1
  Heater Switch2/1 -> Math Function1/1
  Math Function1/1 -> Heater Switch3/2
  Constant3/1 -> Heater Switch3/1
  Subtract1/1 -> Iinst/1, Solar/1
  Constant4/1 -> Subtract1/1
  Heater Switch3/1 -> Subtract1/2
